simulink model "ofdmBAsic"  (Simulink 7.9)
settings: Solver=FixedStepDiscrete  StartTime=0.0  StopTime=100  RelTol=1e-3
model workspace (MATLAB code in the model file):
  | Symbols_per_Frame=45;
undefined symbols (not defined in the file or in its folder): j
libraries: commcnvcod2 x2, dspxfrm3 x2, commdigbbndam3 x2, commchan3 x1, commrandsrc2 x1, commsink2 x1, commutil2 x1
settings Model: Creator=admin  LastModifiedBy=ArunKB

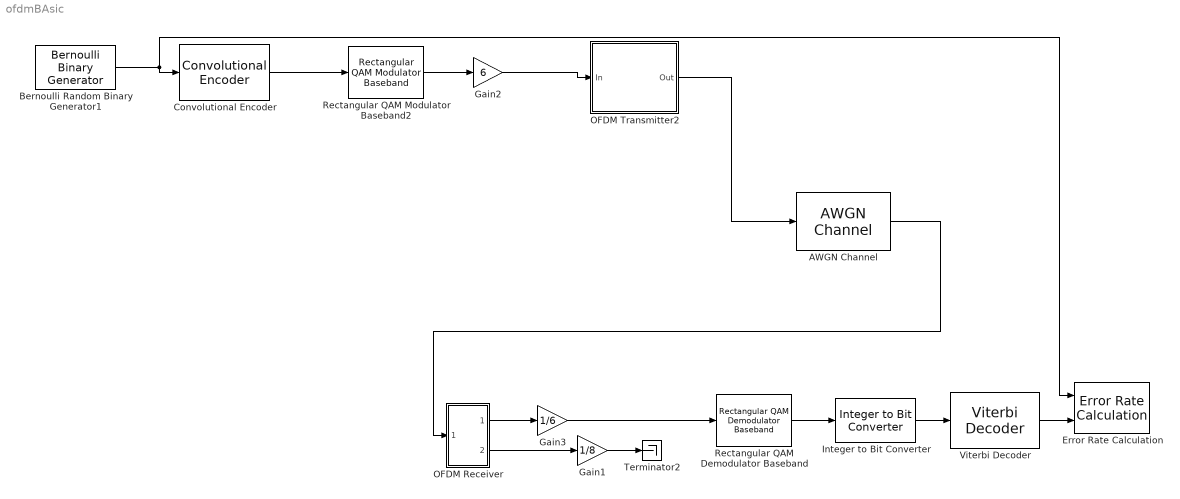
== system ofdmBAsic ==
  AWGN Channel : commchan3/AWGN Channel  InputProcessing=Columns as channels (frame based)  seed=54  noiseMode="Signal to noise ratio  (SNR)"  EbNodB=10  EsNodB=10  SNRdB=SNRvalue  bitsPerSym=1  Ps=1  Tsym=1  variance=1
  Bernoulli Random Binary Generator1 : commrandsrc2/Bernoulli Binary Generator  P=0.5  seed=658  Ts=.001  frameBased=on  sampPerFrame=45  orient=off  outDataType=double
  Convolutional Encoder : commcnvcod2/Convolutional Encoder  trellis=poly2trellis(7, [171 133])  opMode=Truncated (reset every frame)  DelayedResetAction=off  hasIniStPort=off  hasFinStPort=off  usePuncVector=off  punctureVector=[1; 1; 0; 1; 0; 1]  reset=Unused parameter value
  Error Rate Calculation : commsink2/Error Rate Calculation  N=0  st_delay=0  cp_mode=Entire frame  subframe=[]  PMode=Workspace  WsName=ErrorVec  RsMode2=off  stop=off  numErr=100  maxBits=1e6
  Gain1 : Gain  Gain=1/8
  Gain2 : Gain  Gain=6  SaturateOnIntegerOverflow=on  OutDataTypeStr=Inherit: Same as input  ParamDataTypeStr=Inherit: Same as input
  Gain3 : Gain  Gain=1/6  SaturateOnIntegerOverflow=on  OutDataTypeStr=Inherit: Same as input  ParamDataTypeStr=Inherit: Same as input
  Integer to Bit Converter : commutil2/Integer to Bit Converter  nbits=2  signedInputValues=Unsigned  bitOrder=MSB first  outDtype=Inherit via internal rule
  OFDM Receiver : Subsystem
  OFDM Transmitter2 : Subsystem
      mask Display: disp('OFDM\nTransmitter')
  Rectangular QAM Demodulator Baseband : commdigbbndam3/Rectangular QAM Demodulator Baseband  M=4  PowType=Min. distance between symbols  MinDist=2  AvgPow=1  PeakPow=1  Ph=0  Dec=Binary  Mapping=[0:15]  OutType=Integer  DecType=Hard decision  VarSource=Dialog  Variance=1  outDtype1=Inherit via internal rule  outDtype2=Inherit via internal rule  derotateFactorWordLen=16  denormFactorWordLen=16  prodOutWordLen=32  prodOutRoundingMode=Floor  prodOutOverflowMode=Wrap  sumWordLen=32
  Rectangular QAM Modulator Baseband2 : commdigbbndam3/Rectangular QAM Modulator Baseband  M=4  InType=Bit  Enc=Binary  Mapping=[0:15]  PowType=Min. distance between symbols  MinDist=2  AvgPow=1  PeakPow=1  Ph=0  outDtype=double  outWordLen=16  outUDDataType=sfix(16)  outFracLenMode=Best precision  outFracLen=15
  Terminator2 : Terminator
  Viterbi Decoder : commcnvcod2/Viterbi Decoder  trellis=poly2trellis(7, [171 133])  isPunctured=off  punctureVector=[1; 1; 0; 1; 0; 1]  erasures=off  dectype=Hard decision  runSigValErrCheck=off  nsdecb=4  smWordLength=16  tbdepth=45  opmode=Truncated  reset=off  outDataType=Inherit via internal rule  delayedResetAction=off
  wires:
  Rectangular QAM Modulator Baseband2/1 -> Gain2/1
  Gain2/1 -> OFDM Transmitter2/1(In)
  OFDM Receiver/2(Pilot) -> Gain1/1
  OFDM Receiver/1(Data) -> Gain3/1
  Rectangular QAM Demodulator Baseband/1 -> Integer to Bit Converter/1
  Gain3/1 -> Rectangular QAM Demodulator Baseband/1
  Integer to Bit Converter/1 -> Viterbi Decoder/1
  Bernoulli Random Binary Generator1/1 -> Error Rate Calculation/1, Convolutional Encoder/1
  Gain1/1 -> Terminator2/1
  OFDM Transmitter2/1(Out) -> AWGN Channel/1
  AWGN Channel/1 -> OFDM Receiver/1(input)
  Convolutional Encoder/1 -> Rectangular QAM Modulator Baseband2/1
  Viterbi Decoder/1 -> Error Rate Calculation/2

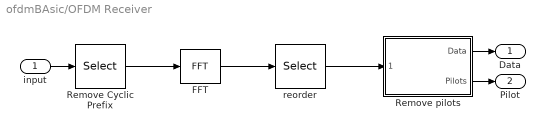
== system ofdmBAsic/OFDM Receiver ==
  input : Inport
  FFT : dspxfrm3/FFT  CompMethod=Table lookup  TableOpt=HYBRID  TableOptActive=Speed  BitRevOrder=off  InheritFFTLength=on  FFTLength=64  RowConvenienceOn=on  FFTImplementation=Auto  SkipNorm=off  firstCoeffDataTypeStr=Inherit: Same word length as input  firstCoeffLastDataTypeStr=Inherit: Same word length as input  outputMin=[]  outputMax=[]  roundingMode=Floor  overflowMode=off
  Remove Cyclic Prefix : Selector  InputPortWidth=80  IndexOptions=Index vector (dialog)  Indices=[17:80]  OutputSizes=1
  Remove pilots : Subsystem
  reorder : Selector  InputPortWidth=64  IndexOptions=Index vector (dialog)  Indices=[33:64 1:32]  OutputSizes=1
  Data : Outport
  Pilot : Outport  Port=2
  wires:
  FFT/1 -> reorder/1
  Remove Cyclic Prefix/1 -> FFT/1
  reorder/1 -> Remove pilots/1("  ")
  Remove pilots/1(Data) -> Data/1
  input/1 -> Remove Cyclic Prefix/1
  Remove pilots/2(Pilots) -> Pilot/1

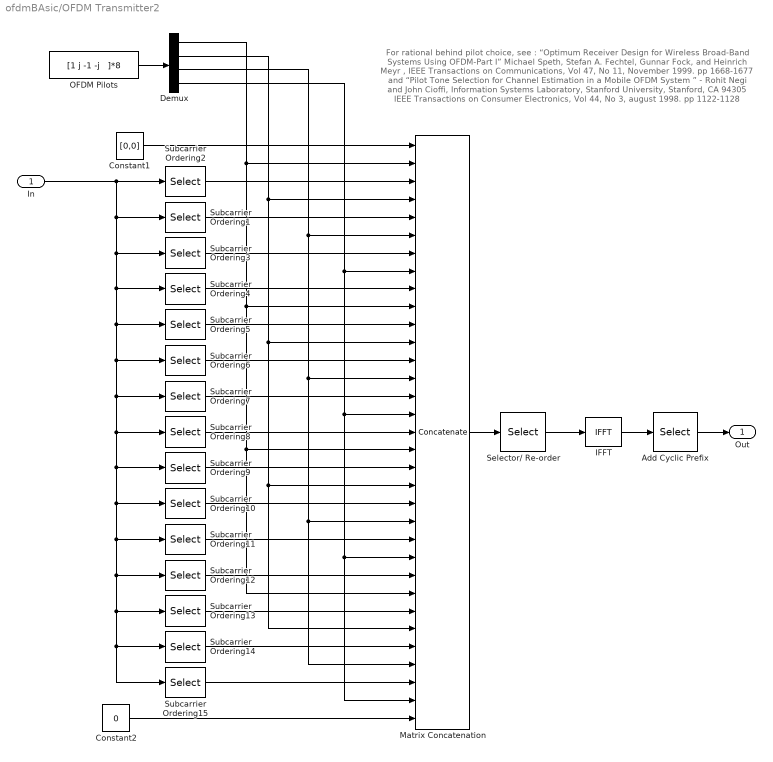
== system ofdmBAsic/OFDM Transmitter2 ==
  note: For rational behind pilot choice, see :
      | “Optimum Receiver Design for Wireless Broad-Band Systems Using OFDM-Part I”
      | Michael Speth, Stefan A. Fechtel, Gunnar Fock, and Heinrich Meyr ,
      |  IEEE Transactions on Communications, Vol 47, No 11, November 1999. pp 1668-1677
      | and
      | “Pilot Tone Selection for Channel Estimation in a Mobile OFDM System ” -
      |  Rohit Negi and John Cioffi, Information Systems Laboratory, Stanford University, Stanford, CA 94305
      | IEEE Transactions on Consumer Electronics, Vol 44, No 3, august 1998. pp 1122-1128
  In : Inport
  Add Cyclic Prefix : Selector  InputPortWidth=64  IndexOptions=Index vector (dialog)  Indices=[49:64 1:64]  OutputSizes=1
  Constant1 : Constant  Value=[0,0]
  Constant2 : Constant  Value=0
  Demux : Demux
  IFFT : dspxfrm3/IFFT  CompMethod=Table lookup  TableOpt=HYBRID  TableOptActive=Speed  BitRevOrder=off  cs_in=off  SkipNorm=on  InheritFFTLength=on  FFTLength=64  mode=Complex  outSamplingMode=Frame based  RowConvenienceOn=on  FFTImplementation=Auto  firstCoeffDataTypeStr=Inherit: Same word length as input  firstCoeffLastDataTypeStr=Inherit: Same word length as input  outputMin=[]  outputMax=[]  roundingMode=Floor  overflowMode=off
  Matrix Concatenation : Concatenate  NumInputs=33  Mode=Multidimensional array
  OFDM Pilots : Constant  Value="[1 j -1 -j   ]*8"
  Selector/ Re-order : Selector  InputPortWidth=64  IndexOptions=Index vector (dialog)  Indices=[33:64 1:32]  OutputSizes=1
  Subcarrier Ordering1 : Selector  InputPortWidth=Symbols_per_Frame  IndexOptions=Index vector (dialog)  Indices=4:6  OutputSizes=1
  Subcarrier Ordering10 : Selector  InputPortWidth=Symbols_per_Frame  IndexOptions=Index vector (dialog)  Indices=28:30  OutputSizes=1
  Subcarrier Ordering11 : Selector  InputPortWidth=Symbols_per_Frame  IndexOptions=Index vector (dialog)  Indices=31:33  OutputSizes=1
  Subcarrier Ordering12 : Selector  InputPortWidth=Symbols_per_Frame  IndexOptions=Index vector (dialog)  Indices=34:36  OutputSizes=1
  Subcarrier Ordering13 : Selector  InputPortWidth=Symbols_per_Frame  IndexOptions=Index vector (dialog)  Indices=37:39  OutputSizes=1
  Subcarrier Ordering14 : Selector  InputPortWidth=Symbols_per_Frame  IndexOptions=Index vector (dialog)  Indices=40:42  OutputSizes=1
  Subcarrier Ordering15 : Selector  InputPortWidth=Symbols_per_Frame  IndexOptions=Index vector (dialog)  Indices=43:45  OutputSizes=1
  Subcarrier Ordering2 : Selector  InputPortWidth=Symbols_per_Frame  IndexOptions=Index vector (dialog)  Indices=1:3  OutputSizes=1
  Subcarrier Ordering3 : Selector  InputPortWidth=Symbols_per_Frame  IndexOptions=Index vector (dialog)  Indices=7:9  OutputSizes=1
  Subcarrier Ordering4 : Selector  InputPortWidth=Symbols_per_Frame  IndexOptions=Index vector (dialog)  Indices=10:12  OutputSizes=1
  Subcarrier Ordering5 : Selector  InputPortWidth=Symbols_per_Frame  IndexOptions=Index vector (dialog)  Indices=13:15  OutputSizes=1
  Subcarrier Ordering6 : Selector  InputPortWidth=Symbols_per_Frame  IndexOptions=Index vector (dialog)  Indices=16:18  OutputSizes=1
  Subcarrier Ordering7 : Selector  InputPortWidth=Symbols_per_Frame  IndexOptions=Index vector (dialog)  Indices=19:21  OutputSizes=1
  Subcarrier Ordering8 : Selector  InputPortWidth=Symbols_per_Frame  IndexOptions=Index vector (dialog)  Indices=22:24  OutputSizes=1
  Subcarrier Ordering9 : Selector  InputPortWidth=Symbols_per_Frame  IndexOptions=Index vector (dialog)  Indices=25:27  OutputSizes=1
  Out : Outport
  wires:
  In/1 -> Subcarrier Ordering14/1, Subcarrier Ordering15/1, Subcarrier Ordering13/1, Subcarrier Ordering12/1, Subcarrier Ordering11/1, Subcarrier Ordering10/1, Subcarrier Ordering9/1, Subcarrier Ordering8/1, Subcarrier Ordering7/1, Subcarrier Ordering6/1, Subcarrier Ordering5/1, Subcarrier Ordering4/1, Subcarrier Ordering3/1, Subcarrier Ordering1/1, Subcarrier Ordering2/1
  IFFT/1 -> Add Cyclic Prefix/1
  Matrix Concatenation/1 -> Selector/ Re-order/1
  Selector/ Re-order/1 -> IFFT/1
  Subcarrier Ordering2/1 -> Matrix Concatenation/3
  Subcarrier Ordering1/1 -> Matrix Concatenation/5
  Subcarrier Ordering3/1 -> Matrix Concatenation/7
  Subcarrier Ordering4/1 -> Matrix Concatenation/9
  Subcarrier Ordering5/1 -> Matrix Concatenation/11
  Subcarrier Ordering6/1 -> Matrix Concatenation/13
  Subcarrier Ordering7/1 -> Matrix Concatenation/15
  Subcarrier Ordering8/1 -> Matrix Concatenation/17
  Subcarrier Ordering9/1 -> Matrix Concatenation/19
  Subcarrier Ordering10/1 -> Matrix Concatenation/21
  Subcarrier Ordering11/1 -> Matrix Concatenation/23
  Subcarrier Ordering12/1 -> Matrix Concatenation/25
  Subcarrier Ordering13/1 -> Matrix Concatenation/27
  Subcarrier Ordering14/1 -> Matrix Concatenation/29
  Subcarrier Ordering15/1 -> Matrix Concatenation/31
  Add Cyclic Prefix/1 -> Out/1
  Constant1/1 -> Matrix Concatenation/1
  Constant2/1 -> Matrix Concatenation/33
  Demux/2 -> Matrix Concatenation/4, Matrix Concatenation/12, Matrix Concatenation/20, Matrix Concatenation/28
  Demux/3 -> Matrix Concatenation/6, Matrix Concatenation/14, Matrix Concatenation/22, Matrix Concatenation/30
  Demux/4 -> Matrix Concatenation/8, Matrix Concatenation/16, Matrix Concatenation/24, Matrix Concatenation/32
  OFDM Pilots/1 -> Demux/1
  Demux/1 -> Matrix Concatenation/26, Matrix Concatenation/18, Matrix Concatenation/10, Matrix Concatenation/2

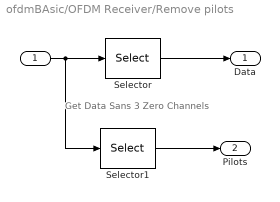
== system ofdmBAsic/OFDM Receiver/Remove pilots ==
  note: Get Data Sans
      | 3 Zero Channels
  "  " : Inport
  Selector : Selector  InputPortWidth=64  IndexOptions=Index vector (dialog)  Indices="[   4:6   8:10  12:14  16:18  20:22  24:26  28:30   32:34  36:38    40:42     44:46   48:50  52:54  56:58   60:62   ]"  OutputSizes=1
  Selector1 : Selector  InputPortWidth=64  IndexOptions=Index vector (dialog)  Indices=[0 1 2 3 4 5 6 7 8 9 10 11 12 13 14 15 ]*4 +3  OutputSizes=1
  Data : Outport
  Pilots : Outport  Port=2
  wires:
  "  "/1 -> Selector/1, Selector1/1
  Selector/1 -> Data/1
  Selector1/1 -> Pilots/1
